simulink model "PD_Monza_simulacion"  (R2025b)
settings: Solver=VariableStepAuto  StartTime=0.0  StopTime=20  RelTol=1e-3
settings Model: Creator=christian  LastModifiedBy=silvi
settings SolverCC: AlgebraicLoopSolver=TrustRegion
settings DataIOCC: ReturnWorkspaceOutputs=off
settings DebuggingCC: UnconnectedInputMsg=warning  UnconnectedOutputMsg=warning  UnconnectedLineMsg=warning  ArithmeticOperatorsInVariantConditions=warning
settings ModelReferenceCC: EnableRefExpFcnMdlSchedulingChecks=on
settings SFSimCC: SimUseLocalCustomCode=off  CustomCodeUndefinedFunction=UseInterfaceOnly
settings RTWCC: RTWUseLocalCustomCode=off  GPUComputeCapability=3.5

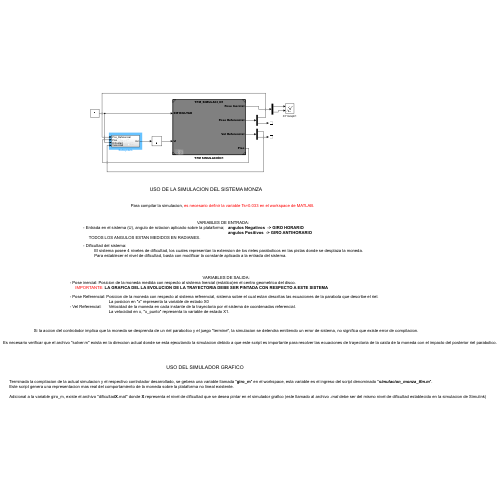
[thumbnail: Simulink's stored preview of the top-level diagram]
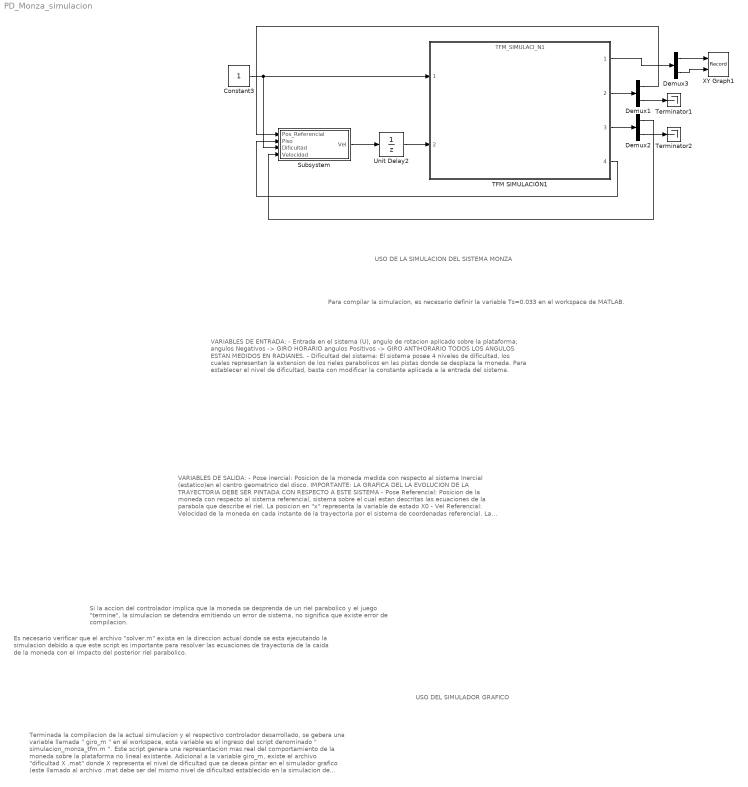
== system PD_Monza_simulacion ==
  note: Es necesario verificar que el archivo "solver.m" exista en la direccion actual donde se esta ejecutando la simulacion debido a que este script es importante para resolver las ecuaciones de trayectoria de la caida de la moneda con el impacto del posterior riel parabolico.
  note: Si la accion del controlador implica que la moneda se desprenda de un riel parabolico y el juego "termine", la simulacion se detendra emitiendo un error de sistema, no significa que existe error de compilacion.
  note: Para compilar la simulacion, es necesario definir la variable Ts=0.033 en el workspace de MATLAB.
  note: VARIABLES DE ENTRADA:
      | - Entrada en el sistema (U), angulo de rotacion aplicado sobre la plataforma; angulos Negativos -> GIRO HORARIO
      | angulos Positivos -> GIRO ANTIHORARIO
      | TODOS LOS ANGULOS ESTAN MEDIDOS EN RADIANES.
      |
      | - Dificultad del sistema:
      | El sistema posee 4 niveles de dificultad, los cuales representan la extension de los rieles parabolicos en las pistas donde se desplaza la moneda.
      | Para establecer el nivel de dificultad, basta con modificar la constante aplicada a la entrada del sistema.
  note: USO DE LA SIMULACION DEL SISTEMA MONZA
  note: VARIABLES DE SALIDA:
      | - Pose inercial: Posicion de la moneda medida con respecto al sistema Inercial (estatico)en el centro geometrico del disco.
      | IMPORTANTE: LA GRAFICA DEL LA EVOLUCION DE LA TRAYECTORIA DEBE SER PINTADA CON RESPECTO A ESTE SISTEMA
      |
      | - Pose Referencial: Posicion de la moneda con respecto al sistema referencial, sistema sobre el cual estan descritas las ecuaciones de la parabola que describe el riel.
      | La posicion en "x" representa la variable de estado X0
      | - Vel Referencial: Velocidad de la moneda en cada instante de la trayectoria por el sistema de coordenadas referencial.
      | La velocidad en x, "x_punto" representa la variable de estado X1.
  note: USO DEL SIMULADOR GRAFICO
  note: Terminada la compilacion de la actual simulacion y el respectivo controlador desarrollado, se gebera una variable llamada " giro_m " en el workspace, esta variable es el ingreso del script denominado " simulacion_monza_tfm.m ".
      | Este script genera una representacion mas real del comportamiento de la moneda sobre la plataforma no lineal existente.
      |
      | Adicional a la variable giro_m, existe el archivo "dificultad X .mat" donde X representa el nivel de dificultad que se desea pintar en el simulador grafico (este llamado al archivo .mat debe ser del mismo nivel de dificultad establecido en la simulacion de Simulink)
  Constant3 : Constant
  Demux1 : Demux  Outputs=2
  Demux2 : Demux  Outputs=2
  Demux3 : Demux  Outputs=2
  Subsystem : Subsystem
  TFM SIMULACIÓN1 : ModelReference  ModelNameDialog=TFM_SIMULACI_N1.slx  UsingDefaultArgumentValue=0,0  SimulationMode=Normal  ModelReferenceVersion=17.1  Gain=0.05  Gain2=0.0223
  Terminator1 : Terminator
  Terminator2 : Terminator
  Unit Delay2 : UnitDelay  SampleTime=-1  HasFrameUpgradeWarning=on
  XY Graph1 : Record  NumPorts=2.0  FileSettingsInternal="{\"entries\":[{\"content\":{\"excelSettings\":{\"content\":{},\"type\":\"Streamout.ExcelSettings\"},\"parquetSettings\":{\"content\":{},\"type\":\"Streamout.ParquetSettings\"}},\"type\":\"Streamout.FileSettingStorage\",\"uuid\":\"\"}],\"packageUris\":[\"http:\\/\\/schema.mathworks.com\\/mf0\\/streamout_blocks\\/R2020a\"],\"version\":\"1.0\"}"  FrameSettings=[0, 0]  Layout=[1 1]  SignalsInternal="{\"entries\":[{\"content\":{\"signals\":[{\"content\":{\"blockPath\":[],\"dimensions\":[1],\"domain\":\"\",\"lineColor\":\"#a2142f\",\"plots\":[ 1 ],\"port\":1,\"sid\":[\"\"],\"signalID\":1,\"signalName\":\"Demux3:1\"},\"type\":\"RecordBlkView.Signal\",\"uuid\":\"\"},{\"content\":{\"blockPath\":[],\"dimensions\":[1],\"domain\":\"\",\"lineColor\":\"#139fff\",\"plots\":[ 1 ],\"port\":2,\"sid\":[\"\"],\"signalID\":2,\"signalName\":\"Demux3:2\"},\"type\":\"RecordBlkView.Signal\",\"uuid\":\"\"}]},\"type\":\"RecordBlkView.InputSignals\",\"uuid\":\"\"}],\"packageUris\":[\"http:\\/\\/schema.mathworks.com\\/mf0\\/streamout_blocks\\/R2020a\"],\"version\":\"1.0\"}"  VisualizationBindings="{\"xyplotplugin\":{\"info\":[{\"series\":[{\"bindingParametersList\":[{\"parameter\":\"X-Axis\",\"signalID\":1,\"signalName\":\"Demux3:1\"},{\"parameter\":\"Y-Axis\",\"signalID\":2,\"signalName\":\"Demux3:2\"}],\"seriesID\":0}],\"subplotID\":1}]}}"  CompatibilityTag=XY  st=-1
  wires:
  Constant3/1 -> Subsystem/3(Dificultad), TFM SIMULACIÓN1/1
  Demux3/1 -> XY Graph1/1
  TFM SIMULACIÓN1/1 -> Demux3/1
  Demux3/2 -> XY Graph1/2
  TFM SIMULACIÓN1/4 -> Subsystem/2(Piso)
  TFM SIMULACIÓN1/2 -> Demux1/1
  Demux1/1 -> Subsystem/1(Pos_Referencial)
  Demux1/2 -> Terminator1/1
  TFM SIMULACIÓN1/3 -> Demux2/1
  Demux2/2 -> Terminator2/1
  Demux2/1 -> Subsystem/4(Velocidad)
  Subsystem/1(Vel) -> Unit Delay2/1
  Unit Delay2/1 -> TFM SIMULACIÓN1/2

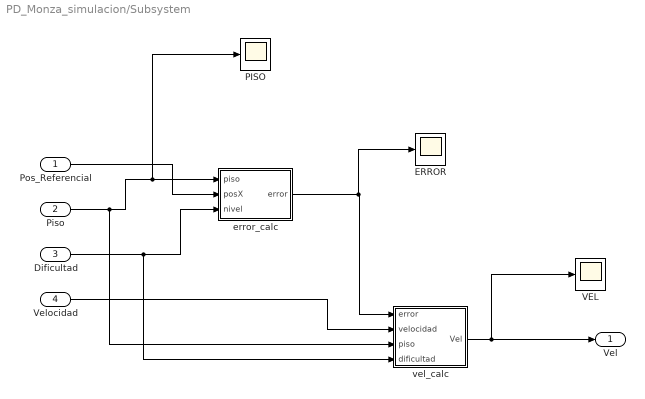
== system PD_Monza_simulacion/Subsystem ==
  Pos_Referencial : Inport
  Piso : Inport  Port=2
  Dificultad : Inport  Port=3
  Velocidad : Inport  Port=4
  ERROR : Scope
      settings: ActiveDisplayYMinimum=-0.51586442560585566  ActiveDisplayYMaximum=0.38010503224030445
  PISO : Scope
      settings: ActiveDisplayYMinimum=0.25000000000000022  ActiveDisplayYMaximum=7.75
  VEL : Scope
      settings: ActiveDisplayYMinimum=-0.36170512224997747  ActiveDisplayYMaximum=0.44511359791313659  DataLoggingVariableName=ScopeData2
  error_calc : MATLAB Function  TreatAsAtomicUnit=on
  vel_calc : MATLAB Function  TreatAsAtomicUnit=on
  Vel : Outport  PortDimensions=1
  wires:
  error_calc/1(error) -> ERROR/1, vel_calc/1(error)
  vel_calc/1(Vel) -> VEL/1, Vel/1
  Piso/1 -> vel_calc/3(piso), PISO/1, error_calc/1(piso)
  Dificultad/1 -> vel_calc/4(dificultad), error_calc/3(nivel)
  Velocidad/1 -> vel_calc/2(velocidad)
  Pos_Referencial/1 -> error_calc/2(posX)

== matlab function PD_Monza_simulacion/Subsystem/vel_calc ==
  data: error input; Vel output; velocidad input; piso input; dificultad input

function Vel = vel_calc(error, velocidad, piso, dificultad)
    Vel = controlador_pid(error, velocidad, dificultad);
end
function Vel = controlador_pid(error, velocidad, dificultad)
    dificultad = max(1, min(4, round(dificultad)));

    ganancias = [3.80, 0.50;
                 3.90, 0.45;
                 7.50, 0.40;
                 5.50, 0.35];

    Kp = ganancias(dificultad, 1);
    Kd = ganancias(dificultad, 2);

    Vel = Kp * error + Kd * velocidad;

    % ---- SATURACION ADAPTATIVA ----
    if abs(error) > 0.10
        Vel = max(-0.32, min(0.32, Vel));  % antes 0.20
    else
        Vel = max(-0.40, min(0.40, Vel));
    end
end

== matlab function PD_Monza_simulacion/Subsystem/error_calc ==
  data: piso input; error output; posX input; nivel input
function error = error_calc(piso, posX, nivel)
    finales = zeros(4, 7, 2);

    % NIVEL 1
    finales(1,:,1) = [0, 0, 0, 0, 0, 0, -0.02554];
    finales(1,:,2) = [0.11429, 0.06857, 0.02286, -0.02286, -0.06857, -0.11429, -0.16035];

    % NIVEL 2
    finales(2,:,1) = [0.06211, -0.04758, 0.04969, -0.04847, 0.04406, -0.05409, -0.02554];
    finales(2,:,2) = [0.11223, 0.06799, 0.02154, -0.02411, -0.06961, -0.11585, -0.16035];

    % NIVEL 3
    finales(3,:,1) = [0.12394, -0.09503, 0.09924, -0.0968, 0.08803, -0.108, -0.02554];
    finales(3,:,2) = [0.10605, 0.06374, 0.01759, -0.02787, -0.07271, -0.12053, -0.16035];

    % NIVEL 4
    finales(4,:,1) = [0.12394, 0.14224, 0.14851, 0.14488, 0.1318, -0.108, -0.02554];
    finales(4,:,2) = [0.10605, 0.05771, 0.01102, -0.03412, -0.07789, -0.12053, -0.16035];

    end_x = finales(nivel, piso, 1);
    error = posX - end_x;

        if nivel == 2 && piso == 3
        fprintf('PISO 3 NIVEL 2: posX = %.4f, end_x = %.4f, error = %.4f\n', posX, end_x, error);
    end
end
